simulink model "accel_jerk_ctrl"  (R2020b)
settings: Solver=VariableStepAuto  StartTime=0.0  StopTime=10.0  RelTol=1e-3
settings Model: Creator=Ricky  LastModifiedBy=Ricky

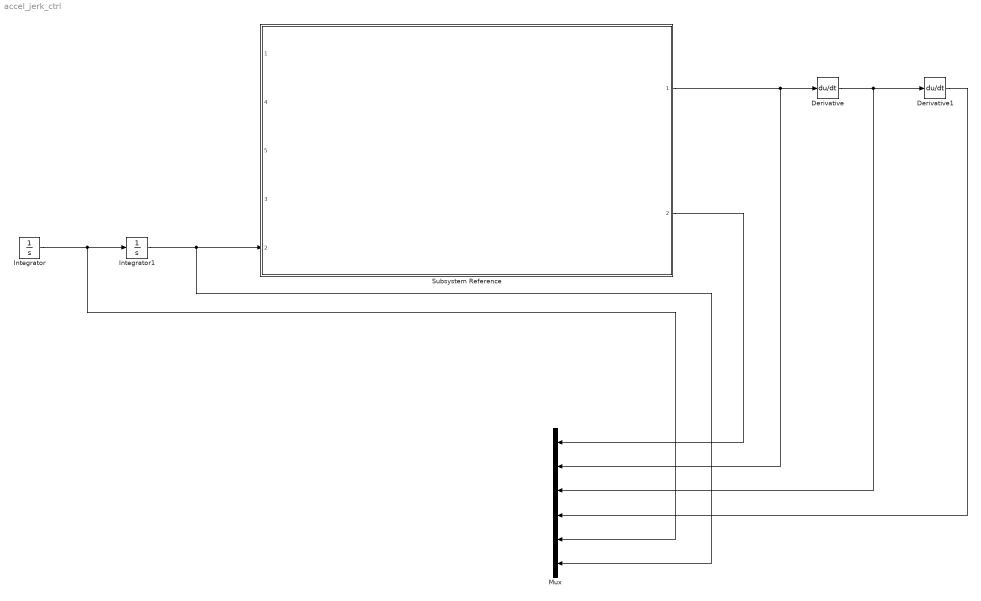
== system accel_jerk_ctrl ==
  Derivative : Derivative
  Derivative1 : Derivative
  Integrator : Integrator
  Integrator1 : Integrator
  Mux : Mux  Inputs=6
  Subsystem Reference : Subsystem  ReferencedSubsystem=quarter_suspension_subsystem
      settings: PortSchema="{\"entries\":[{\"content\":{\"sides\":[{\"content\":{\"connectorIds\":[\"In1\",\"In4\",\"In5\",\"In3\",\"In2\"]},\"type\":\"ConnectorPlacement.EquallySpacedRectSide\",\"uuid\":\"1889bd1a-0e98-4a12-b4d5-f2bbff5a3f70\"},{\"content\":{\"connectorIds\":[\"Out1\",\"Out2\"],\"side\":\"RIGHT\"},\"type\":\"ConnectorPlacement.EquallySpacedRectSide\",\"uuid\":\"a0e9e75d-0456-4878-81af-8c9606bb022b\"},{\"content\":{\"connectorIds\":[],\"side\":\"TOP\"},\"type\":\"ConnectorPlacement.EquallySpacedRectSide\",\"uuid\":\"0af51823-8f8a-4fb0-b1bc-02f03578ba52\"},{\"content\":{\"connectorIds\":[],\"side\":\"HIDDEN\"},\"type\":\"ConnectorPlacement.EquallySpacedRectSide\",\"uuid\":\"54126071-876f-4891-93a6-0d6a6d550f92\"}]},\"type\":\"ConnectorPlacement.EquallySpacedConnector\",\"uuid\":\"ee03e54e-11eb-4a93-aef9-38279e9f3ad5\"}],\"packageUris\":[\"http://schema.mathworks.com/mf0/Connector/R2020b\"],\"version\":\"1.0\"}"
  wires:
  Integrator/1 -> Mux/5, Integrator1/1
  Integrator1/1 -> Mux/6, Subsystem Reference/2
  Subsystem Reference/1 -> Derivative/1, Mux/2
  Subsystem Reference/2 -> Mux/1
  Derivative/1 -> Derivative1/1, Mux/3
  Derivative1/1 -> Mux/4
